simulink model "NXP"  (R2017b)
settings: Solver=FixedStepDiscrete  StartTime=0.0  StopTime=10.0  RelTol=1e-3  EnableMultiTasking=on
libraries: simulink x5, dspswit3 x5, frdmtfcshieldlib x4, frdmkl25zlib x1
settings Model: ModifiedByFormat=The MathWorks Inc.  ExtModeTrigDuration=5  Creator=The MathWorks, Inc.  LastModifiedBy=The MathWorks Inc.
settings DataIOCC: LimitDataPoints=on  SaveFormat=Array
settings OptimizationCC: LifeSpan=1  MaxStackSize=64
settings DebuggingCC: SolverPrmCheckMsg=warning  AllowSymbolicDim=off  SFUnexpectedBacktrackingDiag=warning  SFNoUnconditionalDefaultTransitionDiag=warning  SFExecutionAtInitializationDiag=none
settings HardwareCC: ProdBitPerPointer=32  ProdBitPerSizeT=32  ProdBitPerPtrDiffT=32  ProdLargestAtomicInteger=Long  ProdLargestAtomicFloat=Double  ProdWordSize=32  ProdHWDeviceType=ARM Compatible->ARM Cortex  UseEmbeddedCoderFeatures=off
settings ModelReferenceCC: PropagateSignalLabelsOutOfModel=off
settings RTWCC: SystemTargetFile=ert.tlc  HardwareBoard=NXP FRDM-KL25Z  TemplateMakefile=ert_default_tmf  Toolchain=GNU Tools for ARM Embedded Processors
settings CodeAppCC: StateflowObjectComments=on
settings ERTTargetCC: MultiwordLength=2048  ERTCustomFileBanners=off  SupportContinuousTime=on  SupportNonInlinedSFcns=on  RemoveResetFunc=off  ModelStepFunctionPrototypeControlCompliant=off  ConvertIfToSwitch=off  SuppressUnreachableDefaultCases=off
settings ConfigComp: CovMetricSettings=dw  CovHtmlReporting=on  CovSaveCumulativeToWorkspaceVar=on  CovSaveSingleToWorkspaceVar=on  CovExternalEMLEnable=off  CovSFcnEnable=off

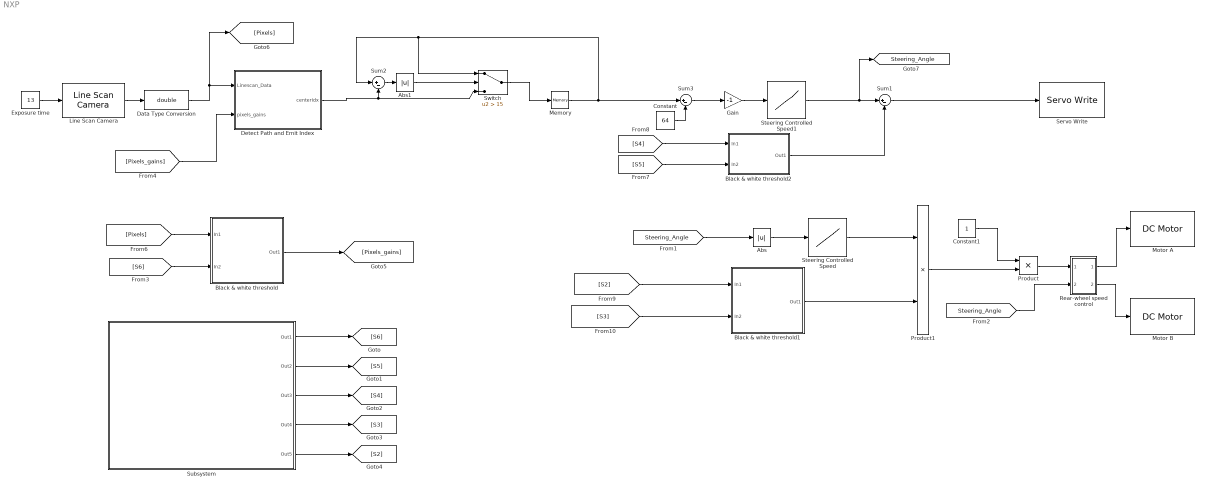
== system NXP ==
  Abs : Abs
  Abs1 : Abs
  Black & white threshold : Subsystem
  Black & white threshold1 : Subsystem
  Black & white threshold2 : Subsystem
  Constant : Constant  Value=64
  Constant1 : Constant
  Data Type Conversion : DataTypeConversion  OutDataTypeStr=double
  Detect Path and Emit Index : MATLAB Function  TreatAsAtomicUnit=on
  Exposure time : Constant  Value=13
  Gain : Gain  Gain=-1
  Line Scan Camera : frdmtfcshieldlib/Line Scan Camera  CameraHeader=0  SampleTime=0.02
      settings: SourceProductName=Simulink Coder Support Package for NXP FRDM-KL25Z Board  SourceProductBaseCode=EC_FREEDOM_BOARD
  Memory : Memory  InitialCondition=64  InheritSampleTime=on
  Motor A : frdmtfcshieldlib/DC Motor  WhichMotor=A
      settings: SourceProductName=Simulink Coder Support Package for NXP FRDM-KL25Z Board  SourceProductBaseCode=EC_FREEDOM_BOARD
  Motor B : frdmtfcshieldlib/DC Motor  WhichMotor=B
      settings: SourceProductName=Simulink Coder Support Package for NXP FRDM-KL25Z Board  SourceProductBaseCode=EC_FREEDOM_BOARD
  Product : Product
  Product1 : Product
  Rear-wheel speed control : Subsystem
  Servo Write : frdmtfcshieldlib/Servo Write  WhichServo=0  minAngle=-30  maxAngle=30
      settings: SourceProductName=Simulink Coder Support Package for NXP FRDM-KL25Z Board  SourceProductBaseCode=EC_FREEDOM_BOARD
  Steering Controlled Speed : Lookup_n-D  NumberOfTableDimensions=1  BreakpointsForDimension1=[0 1 20 30]  Table=[1 0.9 0.6 0.4]  ExtrapMethod=Clip  UseLastTableValue=on  InternalRulePriority=Speed  RndMeth=Simplest  InputSameDT=on
  Steering Controlled Speed1 : Lookup_n-D  NumberOfTableDimensions=1  BreakpointsForDimension1=[-20 -10 -1 1 10 20]  Table=[-30 -8 0 0 8 30]  ExtrapMethod=Clip  UseLastTableValue=on  InternalRulePriority=Speed  RndMeth=Simplest  InputSameDT=on
  Subsystem : Subsystem
  Sum1 : Sum  Inputs=|+-
  Sum2 : Sum  Inputs=|+-
  Sum3 : Sum  Inputs=|+-
  Switch : Switch  Criteria=u2 > Threshold  Threshold=15
  tag scope: Steering_Angle=global
  wires:
  [Pixels_gains] -> Detect Path and Emit Index/2(pixels_gains)
  Black & white threshold/1(Out1) -> [Pixels_gains]
  Sum1/1 -> Servo Write/1
  Subsystem/1(Out1) -> [S6]
  [S2] -> Black & white threshold1/1(In1)
  Subsystem/2(Out2) -> [S5]
  Subsystem/5(Out5) -> [S2]
  [S3] -> Black & white threshold1/2(In2)
  [Steering_Angle] -> Rear-wheel speed control/2(In2)
  [S6] -> Black & white threshold/2(In2)
  Rear-wheel speed control/1(Out1) -> Motor A/1
  [S4] -> Black & white threshold2/1(In1)
  Subsystem/3(Out3) -> [S4]
  Black & white threshold1/1(Out1) -> Product1/2
  [S5] -> Black & white threshold2/2(In2)
  Subsystem/4(Out4) -> [S3]
  Abs/1 -> Steering Controlled Speed/1
  Steering Controlled Speed/1 -> Product1/1
  Rear-wheel speed control/2(Out2) -> Motor B/1
  Exposure time/1 -> Line Scan Camera/1
  Product1/1 -> Product/2
  Constant1/1 -> Product/1
  [Pixels] -> Black & white threshold/1(In1)
  [Steering_Angle] -> Abs/1
  Product/1 -> Rear-wheel speed control/1(In1)
  Line Scan Camera/1 -> Data Type Conversion/1
  Data Type Conversion/1 -> Detect Path and Emit Index/1(Linescan_Data), [Pixels]
  Black & white threshold2/1(Out1) -> Sum1/2
  Detect Path and Emit Index/1(centerIdx) -> Switch/3, Sum2/2
  Sum2/1 -> Abs1/1
  Abs1/1 -> Switch/2
  Switch/1 -> Memory/1
  Constant/1 -> Sum3/2
  Memory/1 -> Sum3/1, Sum2/1, Switch/1
  Sum3/1 -> Gain/1
  Gain/1 -> Steering Controlled Speed1/1
  Steering Controlled Speed1/1 -> [Steering_Angle], Sum1/1

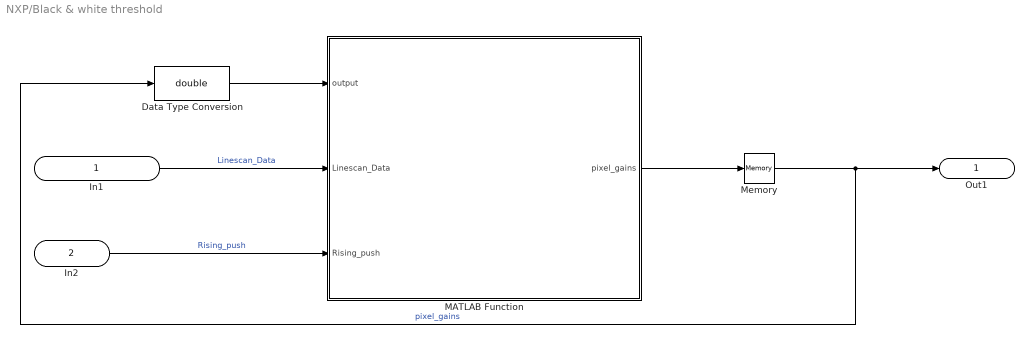
== system NXP/Black & white threshold ==
  In1 : Inport
  In2 : Inport  Port=2
  Data Type Conversion : DataTypeConversion  OutDataTypeStr=double
  MATLAB Function : MATLAB Function  TreatAsAtomicUnit=on
  Memory : Memory  InitialCondition=1  InheritSampleTime=on
  Out1 : Outport
  wires:
  In1/1 -> MATLAB Function/2(Linescan_Data)  "Linescan_Data"
  MATLAB Function/1(pixel_gains) -> Memory/1
  Memory/1 -> Data Type Conversion/1, Out1/1  "pixel_gains"
  In2/1 -> MATLAB Function/3(Rising_push)  "Rising_push"
  Data Type Conversion/1 -> MATLAB Function/1(output)

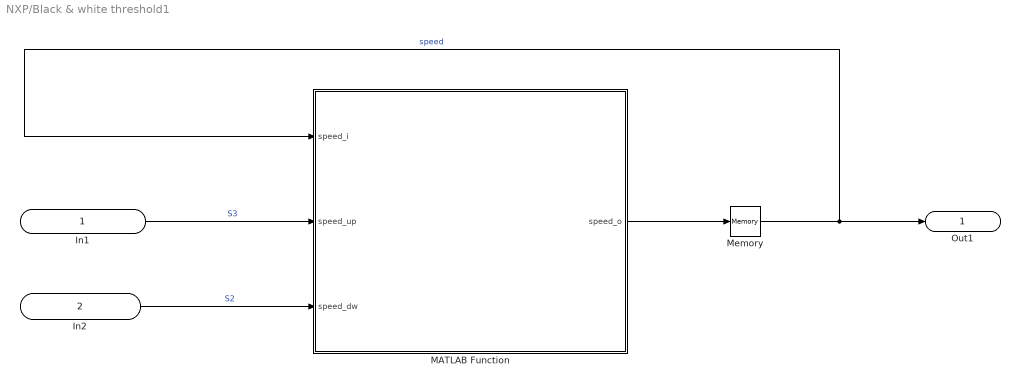
== system NXP/Black & white threshold1 ==
  In1 : Inport
  In2 : Inport  Port=2
  MATLAB Function : MATLAB Function  TreatAsAtomicUnit=on
  Memory : Memory  InheritSampleTime=on
  Out1 : Outport
  wires:
  In1/1 -> MATLAB Function/2(speed_up)  "S3"
  MATLAB Function/1(speed_o) -> Memory/1
  Memory/1 -> MATLAB Function/1(speed_i), Out1/1  "speed"
  In2/1 -> MATLAB Function/3(speed_dw)  "S2"

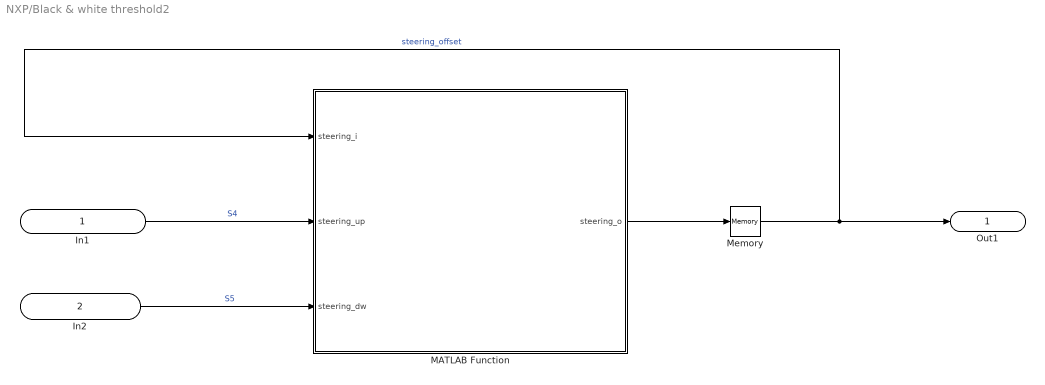
== system NXP/Black & white threshold2 ==
  In1 : Inport
  In2 : Inport  Port=2
  MATLAB Function : MATLAB Function  TreatAsAtomicUnit=on
  Memory : Memory  InheritSampleTime=on
  Out1 : Outport
  wires:
  In1/1 -> MATLAB Function/2(steering_up)  "S4"
  MATLAB Function/1(steering_o) -> Memory/1
  Memory/1 -> MATLAB Function/1(steering_i), Out1/1  "steering_offset"
  In2/1 -> MATLAB Function/3(steering_dw)  "S5"

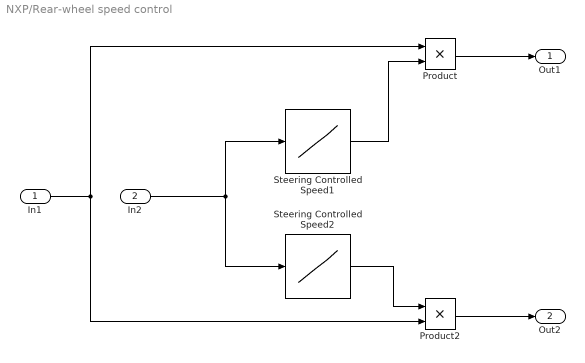
== system NXP/Rear-wheel speed control ==
  In1 : Inport
  In2 : Inport  Port=2
  Product : Product
  Product2 : Product
  Steering Controlled Speed1 : Lookup_n-D  NumberOfTableDimensions=1  BreakpointsForDimension1=[-20 0 20]  Table=[1 1 0.9]  ExtrapMethod=Clip  UseLastTableValue=on  InternalRulePriority=Speed  RndMeth=Simplest  InputSameDT=on
  Steering Controlled Speed2 : Lookup_n-D  NumberOfTableDimensions=1  BreakpointsForDimension1=[-20 0 30]  Table=[0.75 1 1]  ExtrapMethod=Clip  UseLastTableValue=on  InternalRulePriority=Speed  RndMeth=Simplest  InputSameDT=on
  Out1 : Outport
  Out2 : Outport  Port=2
  wires:
  Steering Controlled Speed2/1 -> Product2/1
  In2/1 -> Steering Controlled Speed2/1, Steering Controlled Speed1/1
  In1/1 -> Product2/2, Product/1
  Product/1 -> Out1/1
  Product2/1 -> Out2/1
  Steering Controlled Speed1/1 -> Product/2

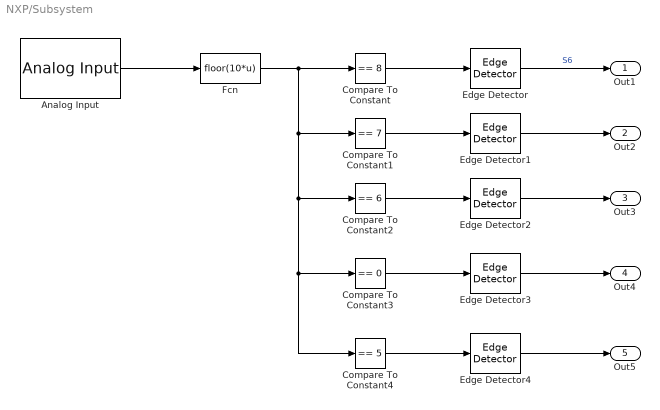
== system NXP/Subsystem ==
  Analog Input : frdmkl25zlib/Analog Input  WhichPin=PTC0  SampleTime=-1
      settings: SourceProductName=Simulink Coder Support Package for NXP FRDM-KL25Z Board  SourceProductBaseCode=EC_FREEDOM_BOARD
  Compare To Constant : simulink/Logic and Bit Operations/Compare To Constant  relop===  const=8  OutDataTypeStr=boolean
  Compare To Constant1 : simulink/Logic and Bit Operations/Compare To Constant  relop===  const=7  OutDataTypeStr=boolean
  Compare To Constant2 : simulink/Logic and Bit Operations/Compare To Constant  relop===  const=6  OutDataTypeStr=boolean
  Compare To Constant3 : simulink/Logic and Bit Operations/Compare To Constant  relop===  const=0  OutDataTypeStr=boolean
  Compare To Constant4 : simulink/Logic and Bit Operations/Compare To Constant  relop===  const=5  OutDataTypeStr=boolean
  Edge Detector{,1..4} (5 alike) : dspswit3/Edge Detector
      settings: SourceProductName=DSP System Toolbox  SourceProductBaseCode=DS
  Fcn : Fcn  Expr=floor(10*u)
  Out1 : Outport  OutDataTypeStr=boolean
  Out2 : Outport  Port=2  OutDataTypeStr=boolean
  Out3 : Outport  Port=3  OutDataTypeStr=boolean
  Out4 : Outport  Port=4  OutDataTypeStr=boolean
  Out5 : Outport  Port=5  OutDataTypeStr=boolean
  wires:
  Fcn/1 -> Compare To Constant1/1, Compare To Constant4/1, Compare To Constant3/1, Compare To Constant2/1, Compare To Constant/1
  Edge Detector/1 -> Out1/1  "S6"
  Compare To Constant/1 -> Edge Detector/1
  Edge Detector3/1 -> Out4/1
  Analog Input/1 -> Fcn/1
  Compare To Constant3/1 -> Edge Detector3/1
  Edge Detector2/1 -> Out3/1
  Edge Detector1/1 -> Out2/1
  Edge Detector4/1 -> Out5/1
  Compare To Constant2/1 -> Edge Detector2/1
  Compare To Constant1/1 -> Edge Detector1/1
  Compare To Constant4/1 -> Edge Detector4/1

== matlab function NXP/Black & white threshold/MATLAB Function ==
  data: output input; pixel_gains output; Linescan_Data input; Rising_push input
function pixel_gains = Correction_pixels(output, Linescan_Data, Rising_push)

% We suppose that the camera cannot see both black edges
pixel_gains = Linescan_Data;

if Rising_push == 0
   pixel_gains = output;
else
   ref = Linescan_Data(64);
   pixel_gains = ref./Linescan_Data;
end

== matlab function NXP/Detect Path and Emit Index ==
  data: centerIdx output single; Linescan_Data input; pixels_gains input
function centerIdx = CenterIdx(Linescan_Data,pixels_gains)
% function centerIdx = CenterIdx(Linescan_Data)


First_Edge=single(2);
Second_Edge=single(127);

Corrected_pixels=pixels_gains.*Linescan_Data;

Half_Value=0.9*max(Corrected_pixels);

%Find the First Edge 
for i=64:-1:3
    if Corrected_pixels(i)<Half_Value
        First_Edge=single(i);
        break;
    end
end
for i=64:1:126
    if Corrected_pixels(i)< Half_Value
        Second_Edge=single(i);
        break;
    end
end

centerIdx=floor((Second_Edge+First_Edge)/2);

% Stop=0;
% cmpt=0;
% 
% Logical_pixels=Corrected_pixels>Half_Value;
% for i=10:118
%     if Logical_pixels(i)==1 && Logical_pixels(i+1)==0
%         cmpt=cmpt+1;
%     end
% end
% 
% if cmpt==4
%     Stop=1;
% end

%%end  minimum finding algorithm

== matlab function NXP/Black & white threshold2/MATLAB Function ==
  data: steering_i input; steering_o output; steering_up input; steering_dw input
function steering_o = Threshold_Switch(steering_i, steering_up, steering_dw)

if steering_up == 1 
    steering_o = steering_i + 1;
elseif steering_dw == 1
    steering_o = steering_i - 1;
else 
    steering_o = steering_i;
end

== matlab function NXP/Black & white threshold1/MATLAB Function ==
  data: speed_i input; speed_o output; speed_up input; speed_dw input
function speed_o = Threshold_Switch(speed_i, speed_up, speed_dw)

if speed_up == 1 
    speed_o = speed_i + 0.05;
elseif speed_dw == 1 && speed_i >= 0.05
    speed_o = speed_i - 0.05;
else 
    speed_o = speed_i;
end
